simulink model "Basic_model"  (R2020b)
settings: Solver=VariableStepAuto  StartTime=0.0  StopTime=10.0  RelTol=1e-3
settings Model: Creator=Akarsh  LastModifiedBy=Akarsh

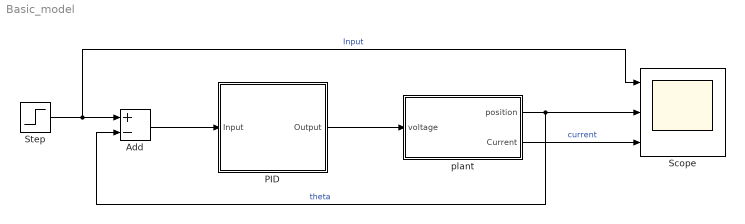
== system Basic_model ==
  Add : Sum  Inputs=+-
  PID : Subsystem
  Scope : Scope  NumInputPorts=3
  Step : Step  Time=2  SampleTime=0
  plant : Subsystem
  wires:
  Step/1 -> Scope/1, Add/1  "Input"
  PID/1(Output) -> plant/1(voltage)
  plant/1(position) -> Add/2, Scope/2  "theta"
  plant/2(Current) -> Scope/3  "current"
  Add/1 -> PID/1("Input ")

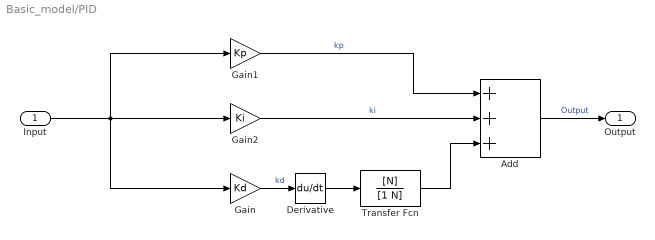
== system Basic_model/PID ==
  "Input " : Inport
  Add : Sum  Inputs=+++
  Derivative : Derivative
  Gain : Gain  Gain=Kd  mask{Kd=23}
  Gain1 : Gain  Gain=Kp  mask{Kp=28, Parameter2=0}
  Gain2 : Gain  Gain=Ki  mask{Ki=895, Parameter2=0}
  Transfer Fcn : TransferFcn  Numerator=[N]  Denominator=[1 N]  mask{N=2182}
  Output : Outport
  wires:
  Gain/1 -> Derivative/1  "kd"
  "Input "/1 -> Gain2/1, Gain/1, Gain1/1
  Gain1/1 -> Add/1  "kp"
  Add/1 -> Output/1  "Output"
  Gain2/1 -> Add/2  "ki"
  Derivative/1 -> Transfer Fcn/1
  Transfer Fcn/1 -> Add/3

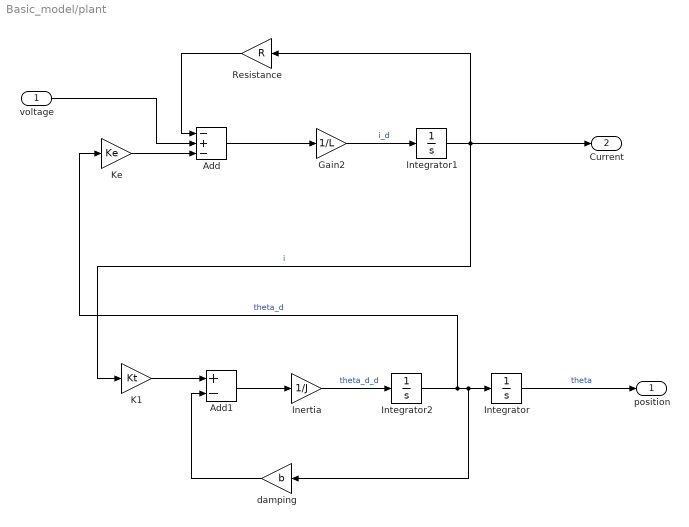
== system Basic_model/plant ==
  voltage : Inport
  Add : Sum  Inputs=-+-
  Add1 : Sum  Inputs=+-
  Gain2 : Gain  Gain=1/L  mask{L=2.75*10^-6}
  Inertia : Gain  Gain=1/J  mask{J=3.22*10^-6}
  Integrator : Integrator
  Integrator1 : Integrator
  Integrator2 : Integrator
  K1 : Gain  Gain=Kt  mask{Kt=0.0274}
  Ke : Gain  Gain=Ke  mask{Ke=0.0274}
  Resistance : Gain  Gain=R  mask{R=4}
  damping : Gain  Gain=b  mask{b=3.5*10^-6}
  position : Outport
  Current : Outport  Port=2
  wires:
  K1/1 -> Add1/1
  Add/1 -> Gain2/1
  voltage/1 -> Add/2
  Gain2/1 -> Integrator1/1  "i_d"
  Resistance/1 -> Add/1
  Integrator1/1 -> Current/1, K1/1, Resistance/1  "i"
  Integrator2/1 -> Integrator/1, damping/1, Ke/1  "theta_d"
  damping/1 -> Add1/2
  Ke/1 -> Add/3
  Add1/1 -> Inertia/1
  Integrator/1 -> position/1  "theta"
  Inertia/1 -> Integrator2/1  "theta_d_d"
